simulink model "trigo_test"  (Simulink 8.4)
settings: Solver=ode45  StartTime=0.0  StopTime=10.0  RelTol=1e-3
settings Model: Creator=arnaud  LastModifiedBy=arnaud

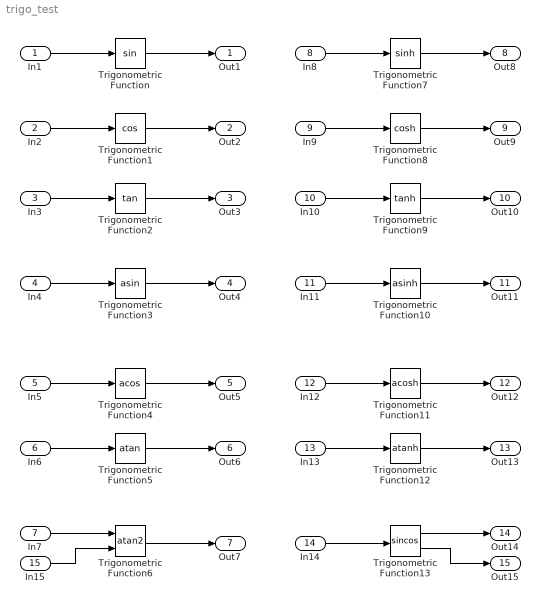
== system trigo_test ==
  In1 : Inport
  In2 : Inport  Port=2
  In3 : Inport  Port=3
  In4 : Inport  Port=4
  In5 : Inport  Port=5
  In6 : Inport  Port=6
  In7 : Inport  Port=7
  In8 : Inport  Port=8
  In9 : Inport  Port=9
  In10 : Inport  Port=10
  In11 : Inport  Port=11
  In12 : Inport  Port=12
  In13 : Inport  Port=13
  In14 : Inport  Port=14
  In15 : Inport  Port=15
  Trigonometric Function : Trigonometry
  Trigonometric Function1 : Trigonometry  Operator=cos
  Trigonometric Function10 : Trigonometry  Operator=asinh
  Trigonometric Function11 : Trigonometry  Operator=acosh
  Trigonometric Function12 : Trigonometry  Operator=atanh
  Trigonometric Function13 : Trigonometry  Operator=sincos
  Trigonometric Function2 : Trigonometry  Operator=tan
  Trigonometric Function3 : Trigonometry  Operator=asin
  Trigonometric Function4 : Trigonometry  Operator=acos
  Trigonometric Function5 : Trigonometry  Operator=atan
  Trigonometric Function6 : Trigonometry  Operator=atan2
  Trigonometric Function7 : Trigonometry  Operator=sinh
  Trigonometric Function8 : Trigonometry  Operator=cosh
  Trigonometric Function9 : Trigonometry  Operator=tanh
  Out1 : Outport
  Out2 : Outport  Port=2
  Out3 : Outport  Port=3
  Out4 : Outport  Port=4
  Out5 : Outport  Port=5
  Out6 : Outport  Port=6
  Out7 : Outport  Port=7
  Out8 : Outport  Port=8
  Out9 : Outport  Port=9
  Out10 : Outport  Port=10
  Out11 : Outport  Port=11
  Out12 : Outport  Port=12
  Out13 : Outport  Port=13
  Out14 : Outport  Port=14
  Out15 : Outport  Port=15
  wires:
  In1/1 -> Trigonometric Function/1
  Trigonometric Function/1 -> Out1/1
  In2/1 -> Trigonometric Function1/1
  Trigonometric Function1/1 -> Out2/1
  In3/1 -> Trigonometric Function2/1
  Trigonometric Function2/1 -> Out3/1
  In4/1 -> Trigonometric Function3/1
  Trigonometric Function3/1 -> Out4/1
  In5/1 -> Trigonometric Function4/1
  Trigonometric Function4/1 -> Out5/1
  In6/1 -> Trigonometric Function5/1
  Trigonometric Function5/1 -> Out6/1
  In7/1 -> Trigonometric Function6/1
  Trigonometric Function6/1 -> Out7/1
  In8/1 -> Trigonometric Function7/1
  Trigonometric Function7/1 -> Out8/1
  In9/1 -> Trigonometric Function8/1
  Trigonometric Function8/1 -> Out9/1
  In10/1 -> Trigonometric Function9/1
  Trigonometric Function9/1 -> Out10/1
  In11/1 -> Trigonometric Function10/1
  Trigonometric Function10/1 -> Out11/1
  In12/1 -> Trigonometric Function11/1
  Trigonometric Function11/1 -> Out12/1
  In13/1 -> Trigonometric Function12/1
  Trigonometric Function12/1 -> Out13/1
  In14/1 -> Trigonometric Function13/1
  Trigonometric Function13/1 -> Out14/1
  In15/1 -> Trigonometric Function6/2
  Trigonometric Function13/2 -> Out15/1
